simulink model "Motor_and_Rotot_Model"  (R2023b)
settings: Solver=VariableStepAuto  StartTime=0.0  StopTime=100  RelTol=1e-3
settings Model: Creator=KOTA-Z  LastModifiedBy=KOTA-Z

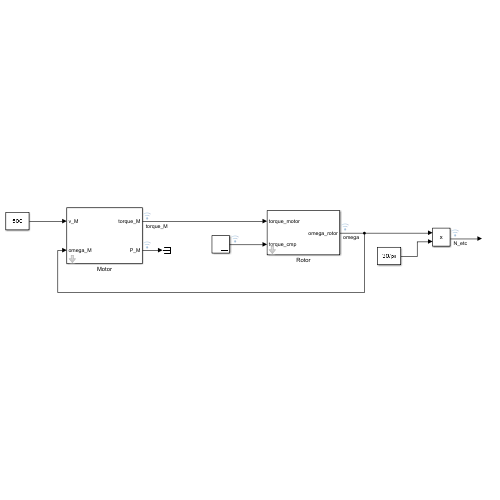
[thumbnail: Simulink's stored preview of the top-level diagram]
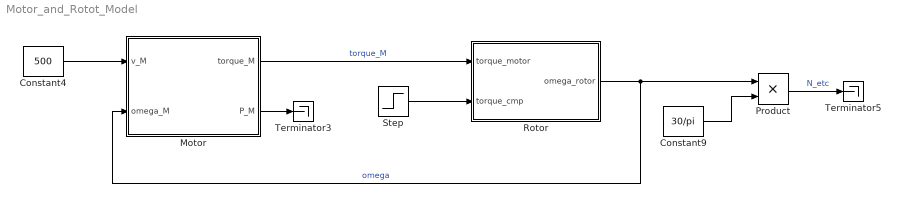
== system Motor_and_Rotot_Model ==
  Constant4 : Constant  Value=500
  Constant9 : Constant  Value=30/pi
  Motor : Subsystem  mask{k_t_M=0.0153, k_e_M=0.0153, R_M=0.82, eta_M=0.98}
      mask prompts: k_t_M "トルク定数 [N*m/A]"; k_e_M "逆起電力係数 [V/(rad/s)]"; R_M "巻線抵抗 [Ω]"; eta_M "モータ機械効率"
      mask DialogControl Parameters Prompt: Motor Parameter
  Product : Product
  Rotor : Subsystem  mask{J_rotor=0.001}
      mask prompts: J_rotor "Inertia [kg*m^2]"
      mask DialogControl Parameters Prompt: Rotor Parameter
  Step : Step  Time=0.1  Before=10  After=9.0643  SampleTime=0
  Terminator3 : Terminator
  Terminator5 : Terminator
  wires:
  Motor/1(torque_M) -> Rotor/1(torque_motor)  "torque_M"
  Constant4/1 -> Motor/1(v_M)
  Motor/2(P_M) -> Terminator3/1
  Rotor/1(omega_rotor) -> Product/1, Motor/2(omega_M)  "omega"
  Product/1 -> Terminator5/1  "N_etc"
  Constant9/1 -> Product/2
  Step/1 -> Rotor/2(torque_cmp)

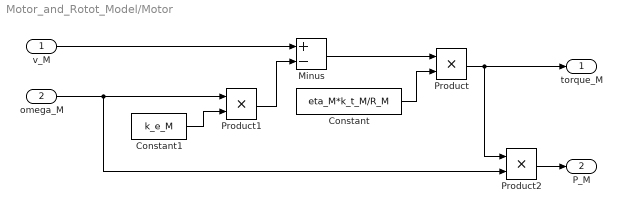
== system Motor_and_Rotot_Model/Motor ==
  v_M : Inport
  omega_M : Inport  Port=2
  Constant : Constant  Value=eta_M*k_t_M/R_M
  Constant1 : Constant  Value=k_e_M
  Minus : Sum  Inputs=+-
  Product : Product
  Product1 : Product
  Product2 : Product
  torque_M : Outport
  P_M : Outport  Port=2
  wires:
  v_M/1 -> Minus/1
  Constant/1 -> Product/2
  Constant1/1 -> Product1/2
  Product1/1 -> Minus/2
  Minus/1 -> Product/1
  omega_M/1 -> Product2/2, Product1/1
  Product/1 -> torque_M/1, Product2/1
  Product2/1 -> P_M/1

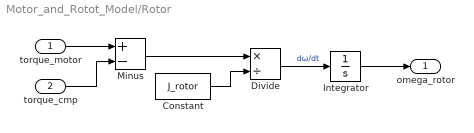
== system Motor_and_Rotot_Model/Rotor ==
  torque_motor : Inport
  torque_cmp : Inport  Port=2
  Constant : Constant  Value=J_rotor
  Divide : Product  Inputs=*/
  Integrator : Integrator
  Minus : Sum  Inputs=+-
  omega_rotor : Outport
  wires:
  Constant/1 -> Divide/2
  Divide/1 -> Integrator/1  "dω/dt"
  Integrator/1 -> omega_rotor/1
  torque_motor/1 -> Minus/1
  Minus/1 -> Divide/1
  torque_cmp/1 -> Minus/2
